simulink model "zad2"  (R2023b)
settings: Solver=VariableStepAuto  StartTime=0.0  StopTime=10.0  RelTol=1e-3
values from neighbouring files (symbols this model uses):
  a = 0.01    [zad2.m]
  k = 0.5    [zad2.m]
  m = 1    [zad2.m]
  x0 = 0.5    [zad2.m]
  x0_poch = 0    [zad2.m]
settings Model: Creator=student  LastModifiedBy=student

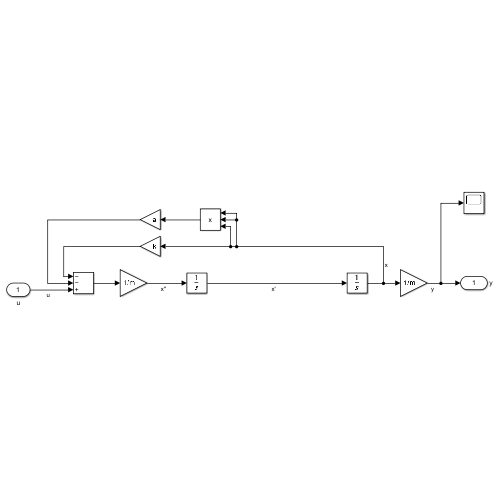
[thumbnail: Simulink's stored preview of the top-level diagram]
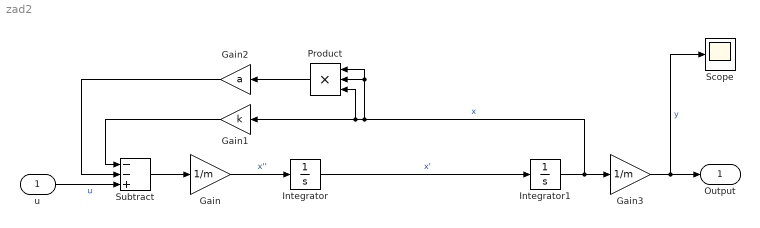
== system zad2 ==
  u : Inport
  Gain : Gain  Gain=1/m
  Gain1 : Gain  Gain=k
  Gain2 : Gain  Gain=a
  Gain3 : Gain  Gain=1/m
  Integrator : Integrator  InitialCondition=x0_poch
  Integrator1 : Integrator  InitialCondition=x0
  Product : Product  Inputs=3
  Scope : Scope
  Subtract : Sum  Inputs=--+
  Output : Outport  SignalName=y
  wires:
  Gain/1 -> Integrator/1  "x''"
  Integrator/1 -> Integrator1/1  "x'"
  Integrator1/1 -> Gain3/1, Gain1/1, Product/3, Product/1, Product/2  "x"
  Subtract/1 -> Gain/1
  Gain1/1 -> Subtract/1
  Product/1 -> Gain2/1
  Gain2/1 -> Subtract/2
  u/1 -> Subtract/3  "u"
  Gain3/1 -> Scope/1, Output/1  "y"
